simulink model "PMSMCurrentControl"  (R2022a)
settings: Solver=ode1  StartTime=0.0  StopTime=10  FixedStep=1e-5  RelTol=1e-3
values from neighbouring files (symbols this model uses):
  A = [0 -Lq  ; Ld 0 ]    [PMSMParameters.m]
  F = 1.57*10.^-3    (= 0.00157)    [PMSMParameters.m]
  J = 5.21*10.^-3    (= 0.00521)    [PMSMParameters.m]
  Kid = Ld*((wne).^2)/Kpd    [PMSMParameters.m]
  Kiq = Lq*((wne).^2)/Kpq    [PMSMParameters.m]
  Kpd = 2*wne*Ld*ceff-Rs    (= 1472.1)    [PMSMParameters.m]
  Kpq = 2*wne*Lq*ceff-Rs    (= 1122.1)    [PMSMParameters.m]
  L = [Ld 0 ; 0 Lq ]    [PMSMParameters.m]
  Ld = 0.3    [PMSMParameters.m]
  Lq = 0.23    [PMSMParameters.m]
  P = 2    [PMSMParameters.m]
  pf = 1.12    [PMSMParameters.m]
  phif = [0 ; pf]    [PMSMParameters.m]
  R = [Rs 0; 0 Rs ]    [PMSMParameters.m]
settings Model: Creator=ZinouAb  LastModifiedBy=habayah
settings ModelReferenceCC: EnableRefExpFcnMdlSchedulingChecks=off
settings RTWCC: Description=Generic Real-Time Target

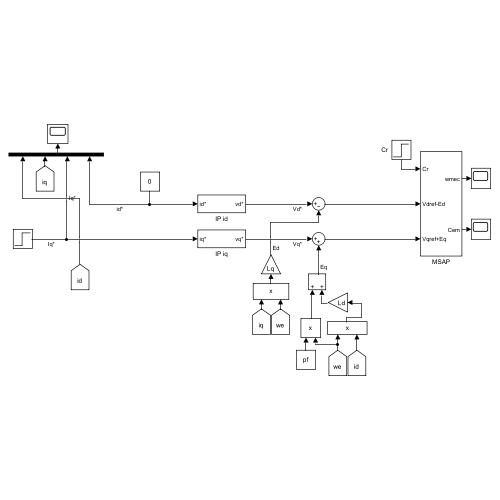
[thumbnail: Simulink's stored preview of the top-level diagram]
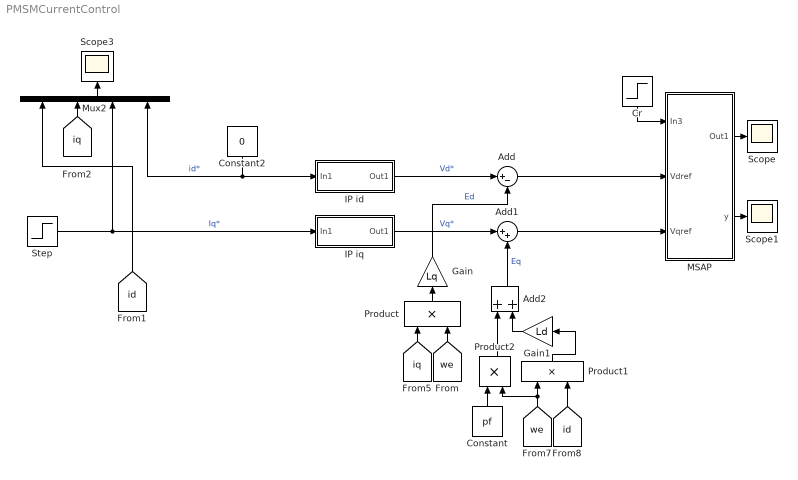
== system PMSMCurrentControl ==
  Add : Sum  Inputs=|+-
  Add1 : Sum  Inputs=|++
  Add2 : Sum
  Constant : Constant  Value=pf
  Constant2 : Constant  Value=0
  Cr : Step  Time=6  Before=0.5  After=3  SampleTime=0
  Gain : Gain  Gain=Lq
  Gain1 : Gain  Gain=Ld
  IP id : Subsystem
  IP iq : Subsystem
  MSAP : Subsystem
  Mux2 : Mux
  Product : Product
  Product1 : Product
  Product2 : Product
  Scope : Scope
  Scope1 : Scope
  Scope3 : Scope
  Step : Step  Time=4  SampleTime=0
  wires:
  IP id/1(Out1) -> Add/1  "Vd*"
  Cr/1 -> MSAP/1(In3)
  MSAP/2(y) -> Scope1/1
  Mux2/1 -> Scope3/1
  MSAP/1(Out1) -> Scope/1
  IP iq/1(Out1) -> Add1/1  "Vq*"
  Constant2/1 -> Mux2/4, IP id/1(In1)  "id*"
  [id] -> Mux2/1
  Step/1 -> IP iq/1(In1), Mux2/3  "Iq*"
  [iq] -> Mux2/2
  Add/1 -> MSAP/2(Vdref)
  Add1/1 -> MSAP/3(Vqref)
  [iq] -> Product/1
  [we] -> Product/2
  Product/1 -> Gain/1
  Gain1/1 -> Add2/2
  Product2/1 -> Add2/1
  Add2/1 -> Add1/2  "Eq"
  Gain/1 -> Add/2  "Ed"
  [we] -> Product2/2, Product1/1
  Constant/1 -> Product2/1
  [id] -> Product1/2
  Product1/1 -> Gain1/1

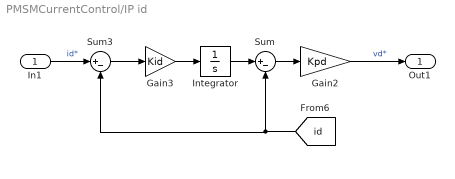
== system PMSMCurrentControl/IP id ==
  In1 : Inport
  Gain2 : Gain  Gain=Kpd
  Gain3 : Gain  Gain=Kid
  Integrator : Integrator
  Sum : Sum  Inputs=|+-
  Sum3 : Sum  Inputs=|+-
  Out1 : Outport
  wires:
  Integrator/1 -> Sum/1
  [id] -> Sum3/2, Sum/2
  Sum/1 -> Gain2/1
  Gain2/1 -> Out1/1  "vd*"
  Gain3/1 -> Integrator/1
  Sum3/1 -> Gain3/1
  In1/1 -> Sum3/1  "id*"

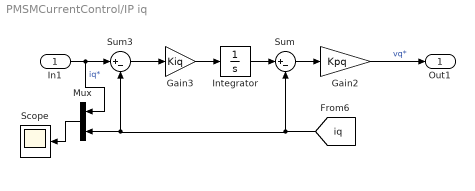
== system PMSMCurrentControl/IP iq ==
  In1 : Inport
  Gain2 : Gain  Gain=Kpq
  Gain3 : Gain  Gain=Kiq
  Integrator : Integrator
  Mux : Mux  Inputs=2
  Scope : Scope
  Sum : Sum  Inputs=|+-
  Sum3 : Sum  Inputs=|+-
  Out1 : Outport
  wires:
  Integrator/1 -> Sum/1
  [iq] -> Mux/2, Sum3/2, Sum/2
  Sum/1 -> Gain2/1
  Gain2/1 -> Out1/1  "vq*"
  Gain3/1 -> Integrator/1
  Sum3/1 -> Gain3/1
  In1/1 -> Mux/1, Sum3/1  "iq*"
  Mux/1 -> Scope/1

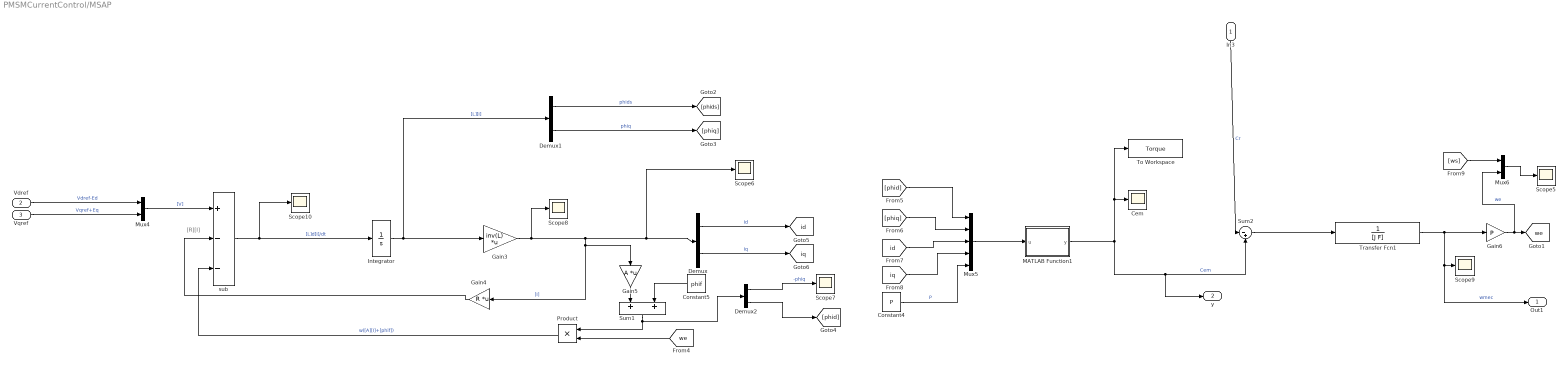
== system PMSMCurrentControl/MSAP ==
  note: [R][I]
  In3 : Inport
  Vdref : Inport  Port=2
  Vqref : Inport  Port=3
  Cem : Scope
  Constant4 : Constant  Value=P
  Constant5 : Constant  Value=phif
  Demux : Demux  Outputs=2
  Demux1 : Demux  Outputs=2
  Demux2 : Demux  Outputs=2
  Gain3 : Gain  Gain=inv(L)  Multiplication=Matrix(K*u)
  Gain4 : Gain  Gain=R  Multiplication=Matrix(K*u)
  Gain5 : Gain  Gain=A  Multiplication=Matrix(K*u)
  Gain6 : Gain  Gain=P
  Integrator : Integrator
  MATLAB Function1 : MATLAB Function  TreatAsAtomicUnit=on
  Mux4 : Mux  Inputs=2
  Mux5 : Mux  Inputs=5
  Mux6 : Mux  Inputs=2
  Product : Product
  Scope{5..10} (6 alike) : Scope
  Sum1 : Sum
  Sum2 : Sum  Inputs=|-+
  To Workspace : ToWorkspace  VariableName=Torque  SaveFormat=Timeseries  SampleTime=-1
  Transfer Fcn1 : TransferFcn  Denominator=[J F]
  sub : Sum  Inputs=+--
  Out1 : Outport
  y : Outport  Port=2
  tag scope: id=global, iq=global, we=global
  wires:
  sub/1 -> Scope10/1, Integrator/1  "[L]d[I]/dt"
  MATLAB Function1/1(y) -> To Workspace/1, Cem/1, y/1, Sum2/2  "Cem"
  Product/1 -> sub/3  "w([A][I]+[phif])"
  Sum2/1 -> Transfer Fcn1/1
  Transfer Fcn1/1 -> Out1/1, Scope9/1, Gain6/1  "wmec"
  Vdref/1 -> Mux4/1  "Vdref-Ed"
  Gain4/1 -> sub/2
  Gain6/1 -> Mux6/2, [we]  "we"
  Demux/2 -> [iq]  "Iq"
  Sum1/1 -> Product/1, Demux2/1
  Demux1/2 -> [phiq]  "phiq"
  Integrator/1 -> Gain3/1, Demux1/1  "[L][I]"
  Mux6/1 -> Scope5/1
  Constant4/1 -> Mux5/5  "P"
  Demux/1 -> [id]  "Id"
  [we] -> Product/2
  Gain5/1 -> Sum1/1
  Gain3/1 -> Gain4/1, Gain5/1, Scope6/1, Demux/1, Scope8/1  "[I]"
  Vqref/1 -> Mux4/2  "Vqref+Eq"
  Mux5/1 -> MATLAB Function1/1(u)
  In3/1 -> Sum2/1  "Cr"
  Constant5/1 -> Sum1/2
  [id] -> Mux5/3
  [iq] -> Mux5/4
  Demux2/2 -> [phid]
  Demux2/1 -> Scope7/1  "-phiq"
  Mux4/1 -> sub/1  "[V]"
  Demux1/1 -> [phids]  "phids"
  [phid] -> Mux5/1
  [phiq] -> Mux5/2
  [ws] -> Mux6/1

== matlab function PMSMCurrentControl/MSAP/MATLAB Function1 ==
  data: u input; y output
function y = CEM(u)

y =(3/2)*u(5)*(u(1)*u(4)-u(2)*u(3));
